simulink model "AmbientMod"  (R2019b)
settings: Solver=FixedStepDiscrete  StartTime=0.0  StopTime=1  FixedStep=1  RelTol=1e-3  EnableMultiTasking=on
libraries: Lib_Turbo_Ambient_TMATS x1
settings Model: Creator=jwchapm2  LastModifiedBy=bhisma
settings DataIOCC: LimitDataPoints=on  SaveFormat=Array  ReturnWorkspaceOutputs=off
settings OptimizationCC: DefaultParameterBehavior=Inlined  ExpressionDepthLimit=2147483647  EfficientTunableParamExpr=on
settings DebuggingCC: UnderspecifiedInitializationDetection=Classic  MergeDetectMultiDrivingBlocksExec=none  SolverPrmCheckMsg=warning  ParameterTunabilityLossMsg=error  StateNameClashWarn=warning  SFUnexpectedBacktrackingDiag=warning  SFNoUnconditionalDefaultTransitionDiag=warning  SFExecutionAtInitializationDiag=none  ArithmeticOperatorsInVariantConditions=warning
settings HardwareCC: ProdBitPerPointer=32  ProdBitPerSizeT=32  ProdBitPerPtrDiffT=32  ProdLargestAtomicFloat=None  ProdIntDivRoundTo=Undefined  ProdEndianess=Unspecified  ProdWordSize=32  ProdHWDeviceType=32-bit Generic  TargetBitPerLong=64  TargetBitPerPointer=64  TargetBitPerSizeT=64  TargetBitPerPtrDiffT=64  TargetLongLongMode=on  TargetIntDivRoundTo=Zero  TargetEndianess=LittleEndian  TargetWordSize=64  TargetHWDeviceType=Generic->MATLAB Host Computer  ProdEqTarget=off
settings ModelReferenceCC: PropagateSignalLabelsOutOfModel=off
settings SFSimCC: SimUseLocalCustomCode=off  MATLABDynamicMemAlloc=off  CustomCodeUndefinedFunction=UseInterfaceOnly
settings RTWCC: SystemTargetFile=ert.tlc  TemplateMakefile=ert_default_tmf  GenerateReport=on  RTWUseLocalCustomCode=off  IncludeHyperlinkInReport=on  LaunchReport=on  GenerateTraceInfo=on  GenerateTraceReport=on  GenerateTraceReportSl=on  GenerateTraceReportSf=on  GenerateTraceReportEml=on
settings CodeAppCC: ForceParamTrailComments=on  IgnoreCustomStorageClasses=off  OperatorAnnotations=on  SimulinkDataObjDesc=on  SFDataObjDesc=on  MATLABFcnDesc=on  InsertBlockDesc=on  StateflowObjectComments=on  MATLABSourceComments=on
settings ERTTargetCC: MultiwordLength=2048  GenerateSampleERTMain=on  InlinedParameterPlacement=NonHierarchical  ERTCustomFileTemplate=example_file_process.tlc
settings ConfigComp: CovMetricSettings=dw  CovHtmlReporting=on  CovSaveCumulativeToWorkspaceVar=on  CovSaveSingleToWorkspaceVar=on  CovExternalEMLEnable=off

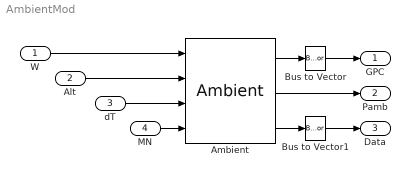
== system AmbientMod ==
  W : Inport
  Alt : Inport  Port=2
  dT : Inport  Port=3
  MN : Inport  Port=4
  Ambient : Lib_Turbo_Ambient_TMATS/Ambient  X_A_AltVec_M=5000*[-1 0 1 2 3 4 5 6 7 8 9 10 12 14 16]  T_A_TsVec_M=[536.51 518.67 500.84 483.03 465.22 447.41 429.62 411.84 394.06 389.97 389.97 389.97 389.97 392.25 397.69]  T_A_PsVec_M=[17.554 14.696 12.228 10.108 8.297 6.759 5.461 4.373 3.468 2.73 2.149 1.692 1.049 0.651 0.406]  AFARc_M=0  X_A_FARVec_M=[0; 0.0050; 0.0100; 0.0150; 0.0200; 0.0250; 0.0300]  T_A_RtArray_M="[0.0686;    0.0686;    0.0686;    0.0686;    0.0686;    0.0686;    0.0686]"  Y_A_TVec_M=[300 10000]  T_A_gammaArray_M=[ 1.4 1.4 1.4 1.4 1.4 1.4 1.4; 1.4 1.4 1.4 1.4 1.4 1.4 1.4]
  Bus to Vector : BusToVector
  Bus to Vector1 : BusToVector
  GPC : Outport
  Pamb : Outport  Port=2
  Data : Outport  Port=3
  wires:
  W/1 -> Ambient/1
  Alt/1 -> Ambient/2
  MN/1 -> Ambient/4
  dT/1 -> Ambient/3
  Ambient/1 -> Bus to Vector/1
  Ambient/2 -> Pamb/1
  Ambient/3 -> Bus to Vector1/1
  Bus to Vector/1 -> GPC/1
  Bus to Vector1/1 -> Data/1
